simulink model "linealizada3"  (Simulink 7.3)
settings: Solver=ode45  StartTime=0.0  StopTime=10.0  RelTol=1e-3
settings Model: Creator=Daniel  LastModifiedBy=Daniel

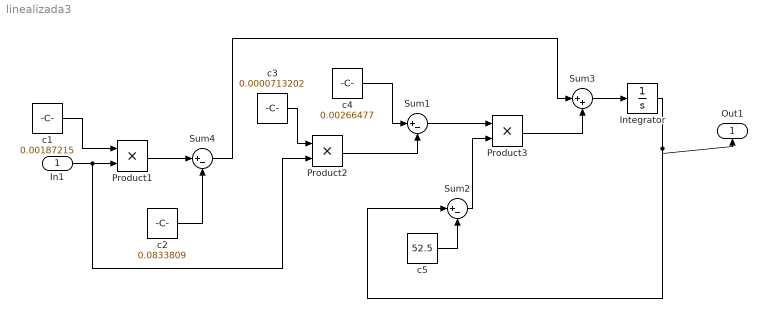
== system linealizada3 ==
  In1 : Inport
  Integrator : Integrator  InitialCondition=10  UpperSaturationLimit=70  LowerSaturationLimit=0.1
  Product1 : Product  SampleTime=0.1  RndMeth=Zero
  Product2 : Product  SampleTime=0.1  RndMeth=Zero
  Product3 : Product  SampleTime=0.1  RndMeth=Zero
  Sum1 : Sum  Inputs=|+-
  Sum2 : Sum  Inputs=|+-
  Sum3 : Sum  Inputs=|++
  Sum4 : Sum  Inputs=|+-
  c1 : Constant  Value=0.00187215
  c2 : Constant  Value=0.0833809
  c3 : Constant  Value=0.0000713202
  c4 : Constant  Value=0.00266477
  c5 : Constant  Value=52.5
  Out1 : Outport
  wires:
  c1/1 -> Product1/1
  In1/1 -> Product1/2, Product2/2
  Product1/1 -> Sum4/1
  c2/1 -> Sum4/2
  c3/1 -> Product2/1
  Product2/1 -> Sum1/2
  c4/1 -> Sum1/1
  c5/1 -> Sum2/2
  Sum2/1 -> Product3/2
  Sum1/1 -> Product3/1
  Product3/1 -> Sum3/2
  Sum4/1 -> Sum3/1
  Sum3/1 -> Integrator/1
  Integrator/1 -> Sum2/1, Out1/1
